simulink model "DrivingSimVR"  (R2020a)
settings: Solver=VariableStepAuto  StartTime=0.0  StopTime=inf  RelTol=1e-3  EnableMultiTasking=on
PostLoadFcn:
  | load position
undefined symbols (not defined in the file or in its folder): serial
libraries: instrumentlib x2, xpcutilitieslib x1, vrlib x1
settings Model: Creator=raoulk  LastModifiedBy=haolee
settings DataIOCC: LimitDataPoints=on  ReturnWorkspaceOutputs=off
settings OptimizationCC: LifeSpan=inf
settings DebuggingCC: AllowSymbolicDim=off  SFUnexpectedBacktrackingDiag=warning  SFNoUnconditionalDefaultTransitionDiag=warning  SFExecutionAtInitializationDiag=none  ArithmeticOperatorsInVariantConditions=warning
settings ModelReferenceCC: PropagateSignalLabelsOutOfModel=off
settings SFSimCC: SimUseLocalCustomCode=off  CustomCodeUndefinedFunction=UseInterfaceOnly
settings RTWCC: RTWUseLocalCustomCode=off
settings CodeAppCC: StateflowObjectComments=on
settings GRTTargetCC: TargetLangStandard=C89/C90 (ANSI)
settings ConfigComp: CovMetricSettings=dw  CovHtmlReporting=on  CovSaveCumulativeToWorkspaceVar=on  CovSaveSingleToWorkspaceVar=on  CovExternalEMLEnable=off

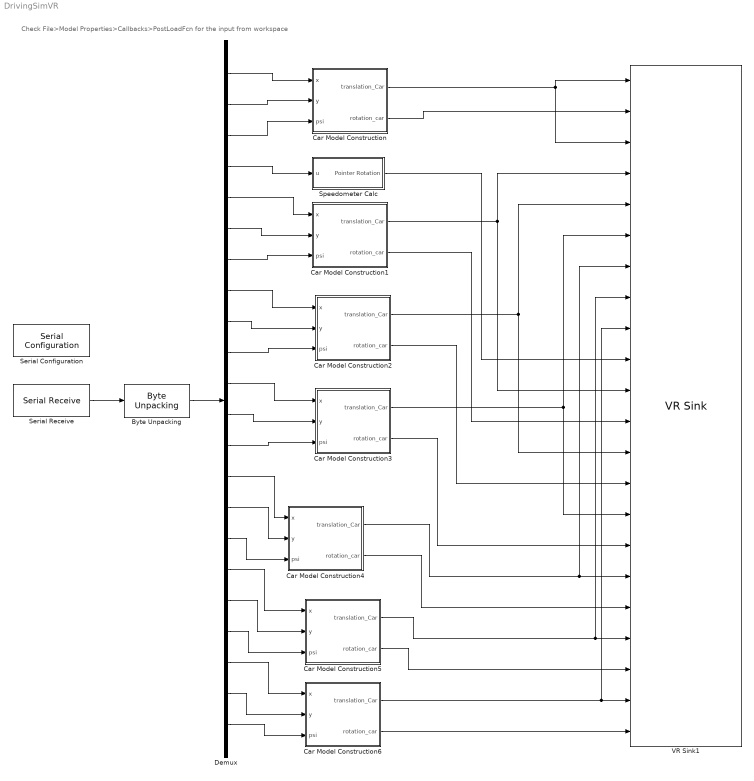
== system DrivingSimVR ==
  note: Check File>Model Properties>Callbacks>PostLoadFcn for the input from workspace
  "Byte Unpacking " : xpcutilitieslib/Byte Unpacking   MaskUnpackedDataTypes={'single'}  MaskUnpackedDataSizes={[22]}  MaskAlignment=1
      settings: SourceProductBaseCode=XP
  Car Model Construction : Subsystem
  Car Model Construction1 : Subsystem
  Car Model Construction2 : Subsystem
  Car Model Construction3 : Subsystem
  Car Model Construction4 : Subsystem
  Car Model Construction5 : Subsystem
  Car Model Construction6 : Subsystem
  Demux : Demux  Outputs=22
  Serial Configuration : instrumentlib/Serial Configuration  Priority=-200000  ComPortMenu=COM4  ComPort=COM4  ObjConstructor=serial('COM4');  BaudRate=115200  DataBits=8  Parity=none  StopBits=1  FlowControl=none  Timeout=20  ByteOrder=LittleEndian
  Serial Receive : instrumentlib/Serial Receive  ComPortMenu=COM4  ComPort=COM4  ObjConstructor=serial('COM4');  Header=s  Terminator=e  DataSize="[88   1]"  DataType=uint8  EnableBlockingMode=on  ActionDataUnavailable=Error  CustomValue=0  SampleTime=0.05
  Speedometer Calc : Subsystem
  VR Sink1 : vrlib/VR Sink  InstantiateOnLoad=on  SampleTime=0.05  ViewEnable=on  RemoteChange=off  RemoteView=off  FieldsWritten=Vehicle1.translation.3.1.1.double#Car_Lotus1.rotation.4.1.1.double#Object1.translation.3.1.1.double#Object2.translation.3.1.1.double#Object3.translation.3.1.1.double#Object4.translation.3.1.1.double#Object5.translation.3.1.1.double#Object7.translation.3.1.1.double#Object6.translation.3.1.1.double#Pointer.rotation.4.1.1.double#Vehicle2.translation.3.1.1.double#Car_Lotus2.rotation.4.1.1.double#Vehicle3.translation.3.1.1.double#Car_Lotus3.rotation.4.1.1.double#Vehicle4.translation.3.1.1.double#Car_Lotus4.rotation.4.1.1.double#Vehicle5.translation.3.1.1.double#Car_Lotus5.rotation.4.1.1.double#Vehicle7.translation.3.1.1.double#Car_Lotus7.rotation.4.1.1.double#Vehicle6.translation.3.1.1.double#Car_Lotus6.rotation.4.1.1.double  WorldFileName=path-11052012.wrl  AutoView=on  VideoDimensions=[]  AllowVariableSize=off  FigureProperties="{'Position', 'Name', 'Viewpoint', 'CameraBound', 'CameraDirection', 'CameraPosition', 'CameraUpVector', 'ZoomFactor', 'Antialiasing', 'Headlight', 'Lighting', 'NavPanel', 'Sound', 'StatusBar', 'Stereo3D', 'Stereo3DCameraOffset', 'Stereo3DHIT', 'ToolBar', 'Textures', 'Transparency', 'Triad', 'Wireframe', 'NavZones', 'NavMode', 'NavSpeed', 'CaptureFileFormat', 'CaptureFileName', 'Record2DCompressMethod', 'Record2DCompressQuality', 'Record2D', 'Record2DFileName', 'Record2DFPS'; [1.2157600000000001e+02   3.8389600000000007e+02   5.7600000000000000e+02   3.5000000000000000e+02], '', 'Vehicle1_Behind', 'on', [0.0000000000000000e+00   0.0000000000000000e+00  -1.0000000000000000e+00], [0.0000000000000000e+00   0.0000000000000000e+00   0.0000000000000000e+00], [0.0000000000000000e+00   1.0000000000000000e+00   0.0000000000000000e+00], [1.0000000000000000e+00], 'on', 'on', 'on', 'halfbar', 'on', 'on', 'off', [1.0000000149011612e-01], [0.0000000000000000e+00], 'on', 'on', 'on', 'none', 'off', 'off', 'fly', 'normal', 'tif', '%f_anim_%n.tif', 'auto', [7.5000000000000000e+01], 'off', '%f_anim_%n.avi', 'auto'}"
  wires:
  Serial Receive/1 -> "Byte Unpacking "/1
  Demux/1 -> Car Model Construction/1(x)
  Demux/2 -> Car Model Construction/2(y)
  Demux/3 -> Car Model Construction/3(psi)
  Demux/4 -> Speedometer Calc/1(u)
  Demux/5 -> Car Model Construction1/1(x)
  Demux/6 -> Car Model Construction1/2(y)
  Demux/7 -> Car Model Construction1/3(psi)
  Demux/8 -> Car Model Construction2/1(x)
  Demux/9 -> Car Model Construction2/2(y)
  Demux/10 -> Car Model Construction2/3(psi)
  Demux/11 -> Car Model Construction3/1(x)
  Demux/12 -> Car Model Construction3/2(y)
  Demux/13 -> Car Model Construction3/3(psi)
  Demux/14 -> Car Model Construction4/1(x)
  Demux/15 -> Car Model Construction4/2(y)
  Demux/16 -> Car Model Construction4/3(psi)
  Demux/17 -> Car Model Construction5/1(x)
  Demux/18 -> Car Model Construction5/2(y)
  Demux/19 -> Car Model Construction5/3(psi)
  Demux/20 -> Car Model Construction6/1(x)
  Demux/21 -> Car Model Construction6/2(y)
  Demux/22 -> Car Model Construction6/3(psi)
  "Byte Unpacking "/1 -> Demux/1
  Car Model Construction1/1(translation_Car) -> VR Sink1/4, VR Sink1/11
  Car Model Construction2/1(translation_Car) -> VR Sink1/5, VR Sink1/13
  Car Model Construction3/1(translation_Car) -> VR Sink1/6, VR Sink1/15
  Car Model Construction4/1(translation_Car) -> VR Sink1/7, VR Sink1/17
  Car Model Construction5/1(translation_Car) -> VR Sink1/8, VR Sink1/19
  Car Model Construction6/1(translation_Car) -> VR Sink1/9, VR Sink1/21
  Car Model Construction/1(translation_Car) -> VR Sink1/3, VR Sink1/1
  Car Model Construction/2(rotation_car) -> VR Sink1/2
  Car Model Construction6/2(rotation_car) -> VR Sink1/22
  Car Model Construction5/2(rotation_car) -> VR Sink1/20
  Car Model Construction4/2(rotation_car) -> VR Sink1/18
  Car Model Construction3/2(rotation_car) -> VR Sink1/16
  Car Model Construction2/2(rotation_car) -> VR Sink1/14
  Car Model Construction1/2(rotation_car) -> VR Sink1/12
  Speedometer Calc/1(Pointer Rotation) -> VR Sink1/10

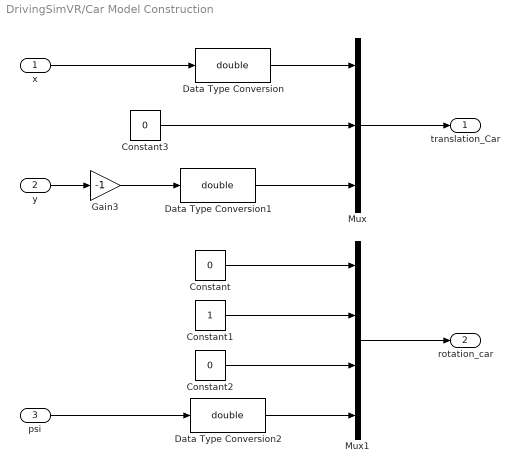
== system DrivingSimVR/Car Model Construction ==
  x : Inport
  y : Inport  Port=2
  psi : Inport  Port=3
  Constant : Constant  Value=0
  Constant1 : Constant
  Constant2 : Constant  Value=0
  Constant3 : Constant  Value=0
  Data Type Conversion : DataTypeConversion  OutDataTypeStr=double
  Data Type Conversion1 : DataTypeConversion  OutDataTypeStr=double
  Data Type Conversion2 : DataTypeConversion  OutDataTypeStr=double
  Gain3 : Gain  Gain=-1
  Mux : Mux  Inputs=3
  Mux1 : Mux
  translation_Car : Outport  VectorParamsAs1DForOutWhenUnconnected=off
  rotation_car : Outport  Port=2  VectorParamsAs1DForOutWhenUnconnected=off
  wires:
  Constant/1 -> Mux1/1
  Constant1/1 -> Mux1/2
  Constant2/1 -> Mux1/3
  Data Type Conversion2/1 -> Mux1/4
  y/1 -> Gain3/1
  psi/1 -> Data Type Conversion2/1
  Constant3/1 -> Mux/2
  Gain3/1 -> Data Type Conversion1/1
  x/1 -> Data Type Conversion/1
  Data Type Conversion1/1 -> Mux/3
  Data Type Conversion/1 -> Mux/1
  Mux/1 -> translation_Car/1
  Mux1/1 -> rotation_car/1

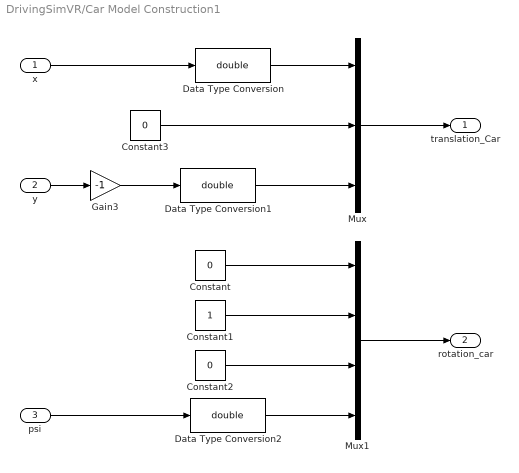
== system DrivingSimVR/Car Model Construction1 ==
  x : Inport
  y : Inport  Port=2
  psi : Inport  Port=3
  Constant : Constant  Value=0
  Constant1 : Constant
  Constant2 : Constant  Value=0
  Constant3 : Constant  Value=0
  Data Type Conversion : DataTypeConversion  OutDataTypeStr=double
  Data Type Conversion1 : DataTypeConversion  OutDataTypeStr=double
  Data Type Conversion2 : DataTypeConversion  OutDataTypeStr=double
  Gain3 : Gain  Gain=-1
  Mux : Mux  Inputs=3
  Mux1 : Mux
  translation_Car : Outport  VectorParamsAs1DForOutWhenUnconnected=off
  rotation_car : Outport  Port=2  VectorParamsAs1DForOutWhenUnconnected=off
  wires:
  Constant/1 -> Mux1/1
  Constant1/1 -> Mux1/2
  Constant2/1 -> Mux1/3
  Data Type Conversion2/1 -> Mux1/4
  y/1 -> Gain3/1
  psi/1 -> Data Type Conversion2/1
  Constant3/1 -> Mux/2
  Gain3/1 -> Data Type Conversion1/1
  x/1 -> Data Type Conversion/1
  Data Type Conversion1/1 -> Mux/3
  Data Type Conversion/1 -> Mux/1
  Mux/1 -> translation_Car/1
  Mux1/1 -> rotation_car/1

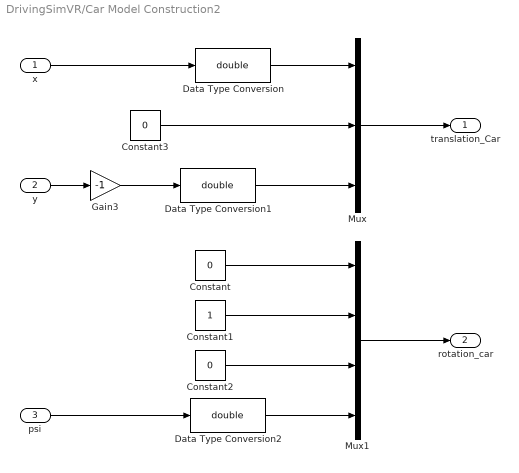
== system DrivingSimVR/Car Model Construction2 ==
  x : Inport
  y : Inport  Port=2
  psi : Inport  Port=3
  Constant : Constant  Value=0
  Constant1 : Constant
  Constant2 : Constant  Value=0
  Constant3 : Constant  Value=0
  Data Type Conversion : DataTypeConversion  OutDataTypeStr=double
  Data Type Conversion1 : DataTypeConversion  OutDataTypeStr=double
  Data Type Conversion2 : DataTypeConversion  OutDataTypeStr=double
  Gain3 : Gain  Gain=-1
  Mux : Mux  Inputs=3
  Mux1 : Mux
  translation_Car : Outport  VectorParamsAs1DForOutWhenUnconnected=off
  rotation_car : Outport  Port=2  VectorParamsAs1DForOutWhenUnconnected=off
  wires:
  Constant/1 -> Mux1/1
  Constant1/1 -> Mux1/2
  Constant2/1 -> Mux1/3
  Data Type Conversion2/1 -> Mux1/4
  y/1 -> Gain3/1
  psi/1 -> Data Type Conversion2/1
  Constant3/1 -> Mux/2
  Gain3/1 -> Data Type Conversion1/1
  x/1 -> Data Type Conversion/1
  Data Type Conversion1/1 -> Mux/3
  Data Type Conversion/1 -> Mux/1
  Mux/1 -> translation_Car/1
  Mux1/1 -> rotation_car/1

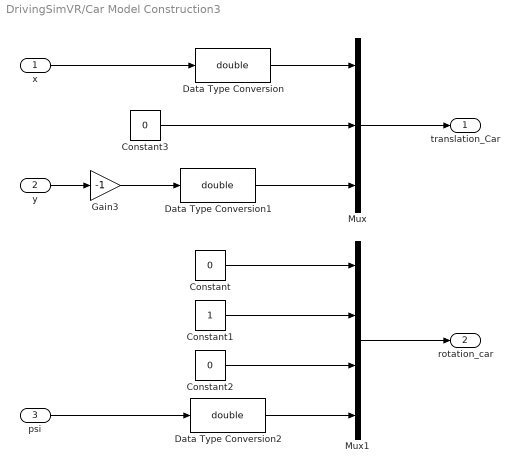
== system DrivingSimVR/Car Model Construction3 ==
  x : Inport
  y : Inport  Port=2
  psi : Inport  Port=3
  Constant : Constant  Value=0
  Constant1 : Constant
  Constant2 : Constant  Value=0
  Constant3 : Constant  Value=0
  Data Type Conversion : DataTypeConversion  OutDataTypeStr=double
  Data Type Conversion1 : DataTypeConversion  OutDataTypeStr=double
  Data Type Conversion2 : DataTypeConversion  OutDataTypeStr=double
  Gain3 : Gain  Gain=-1
  Mux : Mux  Inputs=3
  Mux1 : Mux
  translation_Car : Outport  VectorParamsAs1DForOutWhenUnconnected=off
  rotation_car : Outport  Port=2  VectorParamsAs1DForOutWhenUnconnected=off
  wires:
  Constant/1 -> Mux1/1
  Constant1/1 -> Mux1/2
  Constant2/1 -> Mux1/3
  Data Type Conversion2/1 -> Mux1/4
  y/1 -> Gain3/1
  psi/1 -> Data Type Conversion2/1
  Constant3/1 -> Mux/2
  Gain3/1 -> Data Type Conversion1/1
  x/1 -> Data Type Conversion/1
  Data Type Conversion1/1 -> Mux/3
  Data Type Conversion/1 -> Mux/1
  Mux/1 -> translation_Car/1
  Mux1/1 -> rotation_car/1

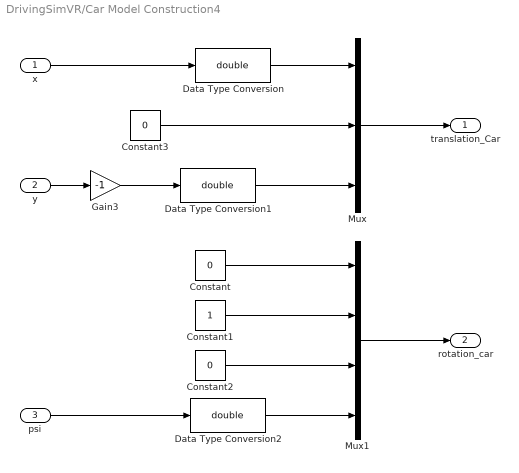
== system DrivingSimVR/Car Model Construction4 ==
  x : Inport
  y : Inport  Port=2
  psi : Inport  Port=3
  Constant : Constant  Value=0
  Constant1 : Constant
  Constant2 : Constant  Value=0
  Constant3 : Constant  Value=0
  Data Type Conversion : DataTypeConversion  OutDataTypeStr=double
  Data Type Conversion1 : DataTypeConversion  OutDataTypeStr=double
  Data Type Conversion2 : DataTypeConversion  OutDataTypeStr=double
  Gain3 : Gain  Gain=-1
  Mux : Mux  Inputs=3
  Mux1 : Mux
  translation_Car : Outport  VectorParamsAs1DForOutWhenUnconnected=off
  rotation_car : Outport  Port=2  VectorParamsAs1DForOutWhenUnconnected=off
  wires:
  Constant/1 -> Mux1/1
  Constant1/1 -> Mux1/2
  Constant2/1 -> Mux1/3
  Data Type Conversion2/1 -> Mux1/4
  y/1 -> Gain3/1
  psi/1 -> Data Type Conversion2/1
  Constant3/1 -> Mux/2
  Gain3/1 -> Data Type Conversion1/1
  x/1 -> Data Type Conversion/1
  Data Type Conversion1/1 -> Mux/3
  Data Type Conversion/1 -> Mux/1
  Mux/1 -> translation_Car/1
  Mux1/1 -> rotation_car/1

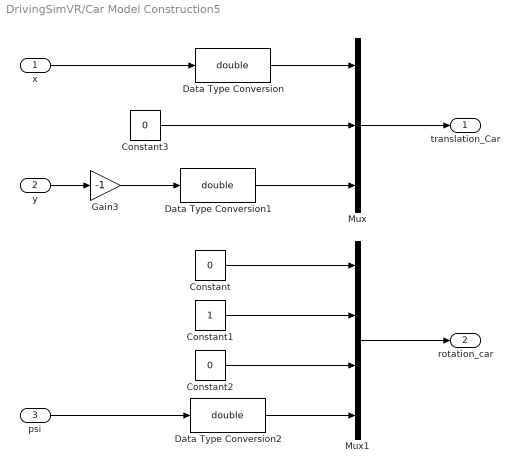
== system DrivingSimVR/Car Model Construction5 ==
  x : Inport
  y : Inport  Port=2
  psi : Inport  Port=3
  Constant : Constant  Value=0
  Constant1 : Constant
  Constant2 : Constant  Value=0
  Constant3 : Constant  Value=0
  Data Type Conversion : DataTypeConversion  OutDataTypeStr=double
  Data Type Conversion1 : DataTypeConversion  OutDataTypeStr=double
  Data Type Conversion2 : DataTypeConversion  OutDataTypeStr=double
  Gain3 : Gain  Gain=-1
  Mux : Mux  Inputs=3
  Mux1 : Mux
  translation_Car : Outport  VectorParamsAs1DForOutWhenUnconnected=off
  rotation_car : Outport  Port=2  VectorParamsAs1DForOutWhenUnconnected=off
  wires:
  Constant/1 -> Mux1/1
  Constant1/1 -> Mux1/2
  Constant2/1 -> Mux1/3
  Data Type Conversion2/1 -> Mux1/4
  y/1 -> Gain3/1
  psi/1 -> Data Type Conversion2/1
  Constant3/1 -> Mux/2
  Gain3/1 -> Data Type Conversion1/1
  x/1 -> Data Type Conversion/1
  Data Type Conversion1/1 -> Mux/3
  Data Type Conversion/1 -> Mux/1
  Mux/1 -> translation_Car/1
  Mux1/1 -> rotation_car/1

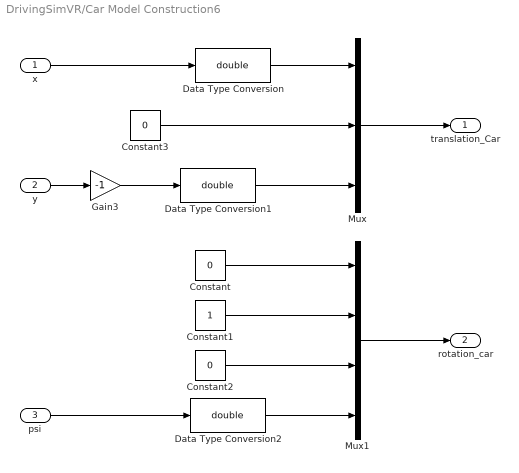
== system DrivingSimVR/Car Model Construction6 ==
  x : Inport
  y : Inport  Port=2
  psi : Inport  Port=3
  Constant : Constant  Value=0
  Constant1 : Constant
  Constant2 : Constant  Value=0
  Constant3 : Constant  Value=0
  Data Type Conversion : DataTypeConversion  OutDataTypeStr=double
  Data Type Conversion1 : DataTypeConversion  OutDataTypeStr=double
  Data Type Conversion2 : DataTypeConversion  OutDataTypeStr=double
  Gain3 : Gain  Gain=-1
  Mux : Mux  Inputs=3
  Mux1 : Mux
  translation_Car : Outport  VectorParamsAs1DForOutWhenUnconnected=off
  rotation_car : Outport  Port=2  VectorParamsAs1DForOutWhenUnconnected=off
  wires:
  Constant/1 -> Mux1/1
  Constant1/1 -> Mux1/2
  Constant2/1 -> Mux1/3
  Data Type Conversion2/1 -> Mux1/4
  y/1 -> Gain3/1
  psi/1 -> Data Type Conversion2/1
  Constant3/1 -> Mux/2
  Gain3/1 -> Data Type Conversion1/1
  x/1 -> Data Type Conversion/1
  Data Type Conversion1/1 -> Mux/3
  Data Type Conversion/1 -> Mux/1
  Mux/1 -> translation_Car/1
  Mux1/1 -> rotation_car/1

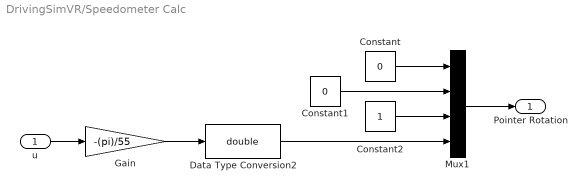
== system DrivingSimVR/Speedometer Calc ==
  u : Inport
  Constant : Constant  Value=0
  Constant1 : Constant  Value=0
  Constant2 : Constant
  Data Type Conversion2 : DataTypeConversion  OutDataTypeStr=double
  Gain : Gain  Gain=-(pi)/55
  Mux1 : Mux
  Pointer Rotation : Outport  VectorParamsAs1DForOutWhenUnconnected=off
  wires:
  Constant/1 -> Mux1/1
  Constant1/1 -> Mux1/2
  Constant2/1 -> Mux1/3
  Data Type Conversion2/1 -> Mux1/4
  Gain/1 -> Data Type Conversion2/1
  u/1 -> Gain/1
  Mux1/1 -> Pointer Rotation/1
